simulink model "Exp_4_3"  (R2024b)
settings: Solver=VariableStepAuto  StartTime=0.0  StopTime=10.0  RelTol=1e-3
settings Model: Creator=Rj Avro Biswas  LastModifiedBy=Rj Avro Biswas

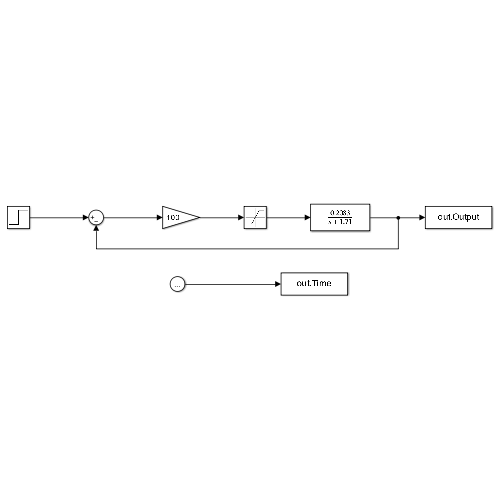
[thumbnail: Simulink's stored preview of the top-level diagram]
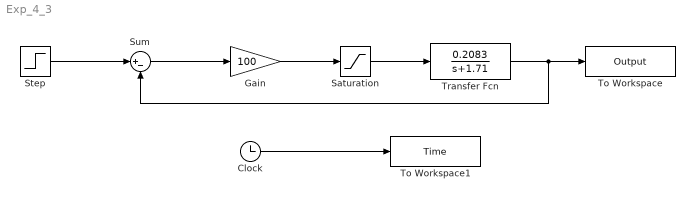
== system Exp_4_3 ==
  Clock : Clock
      settings: Decimation=20
  Gain : Gain  Gain=100
  Saturation : Saturate  UpperLimit=5  LowerLimit=-5
  Step : Step  Time=0  After=10  SampleTime=0
  Sum : Sum  Inputs=|+-
  To Workspace : ToWorkspace  VariableName=Output  SaveFormat=Structure  SampleTime=-1
  To Workspace1 : ToWorkspace  VariableName=Time  SaveFormat=Structure  SampleTime=-1
  Transfer Fcn : TransferFcn  Numerator=0.2083  Denominator=[1 1.71]
  wires:
  Step/1 -> Sum/1
  Sum/1 -> Gain/1
  Gain/1 -> Saturation/1
  Saturation/1 -> Transfer Fcn/1
  Transfer Fcn/1 -> Sum/2, To Workspace/1
  Clock/1 -> To Workspace1/1
